simulink model "simTurboLibMat1_3"  (R2016b)
settings: Solver=VariableStepAuto  StartTime=0.0  StopTime=1  RelTol=1e-3
values from neighbouring files (symbols this model uses):
  variance = 1/(2*r*10^(vectEbNo(i)/10))    [TC_CCSDS_1_2.m]    (also in TC_CCSDS_1_3.m; TC_CCSDS_1_4.m; TC_CCSDS_1_6.m)
undefined symbols (not defined in the file or in its folder): blockLen
libraries: commcnvcod2 x2, commchan3 x1, commrandsrc3 x1, commsink2 x1, commutil2 x1
settings Model: Creator=migm2  LastModifiedBy=migm2

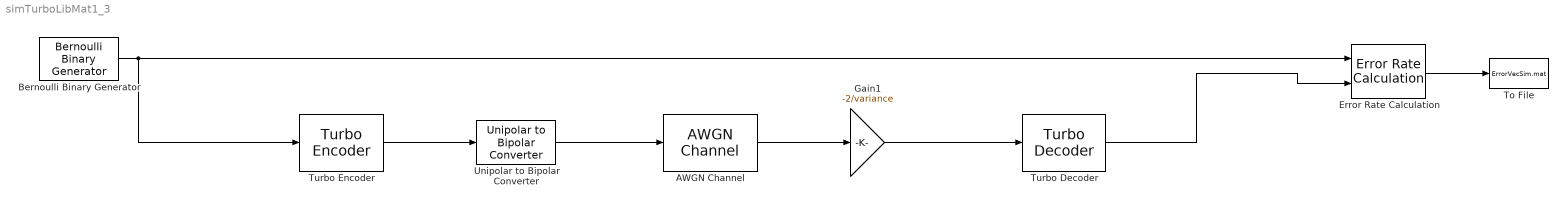
== system simTurboLibMat1_3 ==
  AWGN Channel : commchan3/AWGN Channel  InputProcessing=Columns as channels (frame based)  seed=67  noiseMode=Variance from mask  EbNodB=EbNo  EsNodB=10  SNRdB=10  bitsPerSym=1  Ps=1  Tsym=1/blockLen  variance=variance
  Bernoulli Binary Generator : commrandsrc3/Bernoulli Binary Generator  ProbabilityOfZero=0.5  SeedSource=Parameter  Seed=12345  SampleTime=1/blockLen  SamplesPerFrame=blockLen  OutputDataType=double  SimulateUsing=Interpreted execution
  Error Rate Calculation : commsink2/Error Rate Calculation  N=0  st_delay=0  cp_mode=Entire frame  subframe=[]  PMode=Port  WsName=ErrorVecSim  RsMode2=off  stop=off  numErr=100  maxBits=1e6
  Gain1 : Gain  Gain=-2/variance  SaturateOnIntegerOverflow=on  OutDataTypeStr=Inherit: Same as input  ParamDataTypeStr=Inherit: Same as input
  To File : ToFile  Filename=ErrorVecSim.mat  MatrixName=ErrorVecSim
  Turbo Decoder : commcnvcod2/Turbo Decoder  TrellisStructure=trellis  InterleaverIndicesSource=Property  InterleaverIndices=indInter  Algorithm=True APP  NumScalingBits=3  NumIterations=numIter  SimulateUsing=Interpreted execution
  Turbo Encoder : commcnvcod2/Turbo Encoder  TrellisStructure=trellis  InterleaverIndicesSource=Property  InterleaverIndices=indInter  SimulateUsing=Interpreted execution
  Unipolar to Bipolar Converter : commutil2/Unipolar to Bipolar Converter  M=2  polarity=Negative  dataType=double
  wires:
  Turbo Decoder/1 -> Error Rate Calculation/2
  Bernoulli Binary Generator/1 -> Turbo Encoder/1, Error Rate Calculation/1
  AWGN Channel/1 -> Gain1/1
  Unipolar to Bipolar Converter/1 -> AWGN Channel/1
  Turbo Encoder/1 -> Unipolar to Bipolar Converter/1
  Gain1/1 -> Turbo Decoder/1
  Error Rate Calculation/1 -> To File/1
